simulink model "az4simulinkpreversion"  (R2020a)
settings: Solver=VariableStepAuto  StartTime=0.0  StopTime=10.0  RelTol=1e-3
libraries: cstblocks x1
settings Model: Creator=admin  LastModifiedBy=admin

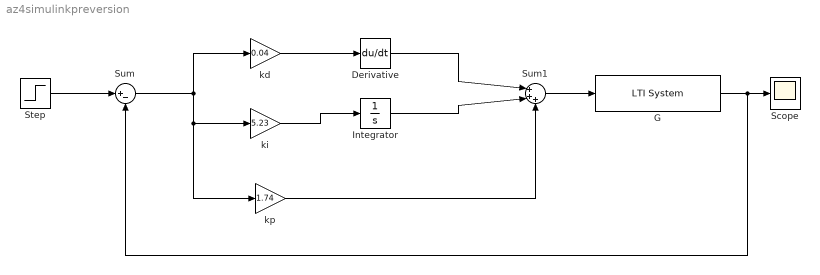
== system az4simulinkpreversion ==
  Derivative : Derivative
  G : cstblocks/LTI System  sys=tf(64.11 , [1 36.42 0])  IC=[]
  Integrator : Integrator
  Scope : Scope
  Step : Step  SampleTime=0
  Sum : Sum  Inputs=|+-
  Sum1 : Sum  Inputs=|+++
  kd : Gain  Gain=0.04
  ki : Gain  Gain=5.23
  kp : Gain  Gain=1.74
  wires:
  Sum/1 -> kp/1, ki/1, kd/1
  kd/1 -> Derivative/1
  ki/1 -> Integrator/1
  Derivative/1 -> Sum1/1
  Integrator/1 -> Sum1/2
  kp/1 -> Sum1/3
  Step/1 -> Sum/1
  Sum1/1 -> G/1
  G/1 -> Sum/2, Scope/1
